simulink model "HostOfSeal"  (R2025a)
settings: Solver=FixedStepDiscrete  StartTime=0.0  StopTime=30  FixedStep=0.025  RelTol=1e-3
model workspace (MATLAB code in the model file + MAT data in the model file):
  | cmdLim = Simulink.Parameter;
  | cmdLim.Value = 15;
  | cmdLim.Description = 'Limit for controlling the maximum surface command angle.';
  | cmdLim.Min = 0;
  | cmdLim.Max = 90;
  | cmdLim.DocUnits = 'deg';
  | 
  | dispGain = Simulink.Parameter;
  | dispGain.Value = 0.75;
  | dispGain.Description = 'Gain applied to the displacement error.';
  | dispGain.Min = 0;
  | dispGain.Max = [];
  | dispGain.DocUnits = 'deg/sec/deg';
  | 
  | dispLim = Simulink.Parameter;
  | dispLim.Value = 30;
  | dispLim.Description = 'Limit for controlling the maximum commanded angle.';
  | dispLim.Min = 0;
  | dispLim.Max = 180;
  | dispLim.DocUnits = 'deg';
  | 
  | intGain = Simulink.Parameter;
  | intGain.Value = 0.5;
  | intGain.Description = 'Gain applied to the integral error.';
  | intGain.Min = 0;
  | intGain.Max = [];
  | intGain.DocUnits = 'deg/sec/deg/sec';
  | 
  | intLim = Simulink.Parameter;
  | intLim.Value = 5;
  | intLim.Description = 'Limit for controlling the maximum commanded angle.';
  | intLim.Min = 0;
  | intLim.Max = 90;
  | intLim.DocUnits = 'deg';
  | 
  | rateGain = Simulink.Parameter;
  | rateGain.Value = 2;
  | rateGain.Description = 'Gain applied to the rate error.';
  | rateGain.Min = 0;
  | rateGain.Max = [];
  | rateGain.DocUnits = 'deg/deg/sec';
  | 
  | rateLim = Simulink.Parameter;
  | rateLim.Value = 6;
  | rateLim.Description = 'Limit for controlling the maximum commanded angle.';
  | rateLim.Min = 0;
  | rateLim.Max = 180;
  | rateLim.DocUnits = 'deg/sec';
  | 
  | hdgGain = Simulink.Parameter;
  | hdgGain.Value = 0.015;
values from neighbouring files (symbols this model uses):
  DriveTs = 100e-6    (= 0.0001)    [simpars.m]
  Jm = 1    [simpars.m]
  KEp = Kt * sqrt(2) / 1.5    [simpars.m]
  Kt = 1    [simpars.m]
  Lm = 1e-3    (= 0.001)    [simpars.m]
  PolePairs = 5    [simpars.m]
  Rm = 1    [simpars.m]
  Vdc = 24    [simpars.m]
undefined symbols (not defined in the file or in its folder): CurrentCommand, DcBusVoltage, EncoderMain, EncoderMainSpeed, Iq, KiSpeed, Kp, KpSpeed, PositionCommand, SpeedCommand, SystemTime
libraries: simulink x1
(part 1 of 2)
Description:
  | This model represents a basic roll axis autopilot with two operating
  | modes; roll attitude hold and heading hold. The mode logic for these
  | modes is external to this model.  The model architecture represents the
  | heading hold mode and basic roll attitude function as referenced models.
  | 
  | The roll attitude control function is a PID controller that uses roll
  | attitude and roll rate feedback to produce an aileron command.  The
  | input to the controller will be either a basic roll angle reference or a
  | roll command to track the desired heading.
settings Model: RequirementInfo={} %GIDa_fe9045fd_0412_4b6e_8206_617cc20e6fde  DataDictionary=SEALGenericTypes_1.sldd  FPTRunName=Active  ModifiedByFormat=The MathWorks, Inc.  Creator=The MathWorks, Inc.  LastModifiedBy=The MathWorks, Inc.
settings SolverCC: AlgebraicLoopSolver=TrustRegion
settings DataIOCC: ExternalInput=xin  SaveFormat=StructureWithTime  SaveOutput=off  SignalLogging=off  DSMLogging=off  SaveTime=off  ReturnWorkspaceOutputs=off
settings OptimizationCC: DefaultParameterBehavior=Inlined  UseDivisionForNetSlopeComputation=on  UseFloatMulNetSlope=on  InlineInvariantSignals=on  ReuseModelBlockBuffer=off  EnhancedBackFolding=on  BooleansAsBitfields=on  PassReuseOutputArgsAs=Individual arguments  ExpressionDepthLimit=2147483647.0  StateBitsets=on  DataBitsets=on  ZeroExternalMemoryAtStartup=off  ZeroInternalMemoryAtStartup=off  NoFixptDivByZeroProtection=on  EfficientFloat2IntCast=on  LifeSpan=inf  MaxStackSize=inf  EfficientTunableParamExpr=on
settings DebuggingCC: SignalRangeChecking=error  ReadBeforeWriteMsg=EnableAllAsError  WriteAfterWriteMsg=EnableAllAsError  WriteAfterReadMsg=EnableAllAsError  AlgebraicLoopMsg=error  ArtificialAlgebraicLoopMsg=error  SaveWithDisabledLinksMsg=error  SaveWithParameterizedLinksMsg=error  CheckExecutionContextPreStartOutputMsg=on  BlockPriorityViolationMsg=error  MaxConsecutiveZCsMsg=warning  SolverPrmCheckMsg=error  InheritedTsInSrcMsg=error  SingleTaskRateTransMsg=error  TasksWithSamePriorityMsg=error  SigSpecEnsureSampleTimeMsg=error  IntegerOverflowMsg=error  ParameterUnderflowMsg=error  ParameterPrecisionLossMsg=none  ParameterTunabilityLossMsg=error  UnderSpecifiedDataTypeMsg=error  UnnecessaryDatatypeConvMsg=warning  VectorMatrixConversionMsg=error  SignalLabelMismatchMsg=error  UnconnectedInputMsg=error  UnconnectedOutputMsg=error  UnconnectedLineMsg=error  SFcnCompatibilityMsg=error  UniqueDataStoreMsg=error  BusObjectLabelMismatch=error  RootOutportRequireBusObject=error  AssertControl=DisableAll  AllowSymbolicDim=off  ModelReferenceIOMismatchMessage=error  UnknownTsInhSupMsg=error  ModelReferenceDataLoggingMessage=error  ModelReferenceSymbolNameMessage=none  StateNameClashWarn=warning  StrictBusMsg=ErrorOnBusTreatedAsVector  NonBusSignalsTreatedAsBus=error  SFInvalidInputDataAccessInChartInitDiag=error  SFTransitionOutsideNaturalParentDiag=error  SFUnreachableExecutionPathDiag=error  SFUndirectedBroadcastEventsDiag=error  SFExecutionAtInitializationDiag=none  IntegerSaturationMsg=error  ArithmeticOperatorsInVariantConditions=warning
settings HardwareCC: ProdBitPerChar=16.0  ProdBitPerInt=16.0  ProdBitPerPointer=32.0  ProdBitPerSizeT=32.0  ProdBitPerPtrDiffT=32.0  ProdLargestAtomicInteger=Integer  ProdLargestAtomicFloat=None  ProdWordSize=16.0  ProdHWDeviceType=Texas Instruments->C2000  TargetHWDeviceType=32-bit Generic
settings ModelReferenceCC: EnableRefExpFcnMdlSchedulingChecks=on  ModelReferenceNumInstancesAllowed=Single  PropagateSignalLabelsOutOfModel=off
settings SFSimCC: SimUseLocalCustomCode=off  MATLABDynamicMemAlloc=off
settings SFSimCC: SimCustomHeaderCode=|
  | #include "CANServer.h"
  | #include "DeviceSetup.h"
settings SFSimCC: SimUserSources=|
  | .\ExternalCode\CANServer.c
  | .\ExternalCode\DeviceSetup.c
settings RTWCC: SystemTargetFile=ert.tlc  GenCodeOnly=on  TemplateMakefile=ert_default_tmf  PostCodeGenCommand=PrepWrapper  GenerateReport=on  RTWVerbose=off  RTWUseLocalCustomCode=off  RTWUseSimCustomCode=on  BuildConfiguration=Faster Runs  IncludeHyperlinkInReport=on  LaunchReport=on  GenerateTraceInfo=on  GenerateTraceReport=on  GenerateTraceReportSl=on  GenerateTraceReportSf=on  GenerateTraceReportEml=on  GenerateCodeMetricsReport=on  GPUComputeCapability=3.5  DLArmComputeVersion=19.05  Description=Embedded Coder
settings RTWCC: CustomHeaderCode=|
  | #include "CANServer.h"
  | #include "DeviceSetup.h"
settings RTWCC: CustomSource=|
  | .\ExternalCode\CANServer.c
  | .\ExternalCode\DeviceSetup.c
settings CodeAppCC: ForceParamTrailComments=on  IgnoreCustomStorageClasses=off  SimulinkDataObjDesc=on  CustomSymbolStrGlobalVar=rt$N$M  CustomSymbolStrType=$N$M  CustomSymbolStrFcn=$N$M$F  CustomSymbolStrMacro=$N$M  InsertBlockDesc=on  ReqsInCode=on
settings ERTTargetCC: ExtModeTransport=0.0  ExtModeStaticAlloc=off  ExtModeMexFile=ext_comm  ExtModeIntrfLevel=Level1  ERTCustomFileTemplate=example_file_process.tlc  ERTFilePackagingFormat=CompactWithDataFile  ConvertIfToSwitch=off  SuppressUnreachableDefaultCases=off  DynamicArrayContainerType=coder::array  UtilityFuncGeneration=Shared location  MultiwordLength=2048.0  GenerateSampleERTMain=on  IncludeMdlTerminateFcn=off  CombineSignalStateStructs=on  SuppressErrorStatus=on  SupportAbsoluteTime=off  SubcomponentCodeInterfacePackaging=Nonreusable function  SupportNonFinite=off  SupportComplex=off
settings ConfigComp: CovScope=ReferencedModels  CovSaveName=covdata_rollAP  CovMetricSettings=dcmtrwe  CovHTMLOptions=-sRT=1 -aTS=1 -bRG=1 -bTC=1 -hTR=1 -nFC=0 -scm=1 -bcm=1 -xEv=0  CovSaveCumulativeToWorkspaceVar=on  CovSaveSingleToWorkspaceVar=on  CovCumulativeVarName=covCumulativeData_rollAP  CovReportOnPause=off  CovExternalEMLEnable=off  CovSFcnEnable=off  DVMaxProcessTime=300.0  DVModelCoverageObjectives=MCDC  DVMaxTestCaseSteps=500.0  DVTestSuiteOptimization=Auto  DVAbsoluteTolerance=1.0e-5  DVDefectChecker=off  DVDetectActiveLogic=on  DVMaxViolationSteps=20.0  DVSaveHarnessModel=on  DVModelReferenceHarness=on  DVHarnessSource=Signal Editor  DVSaveReport=on  DVRebuildModelRepresentation=Always  DVActiveTab=0.0

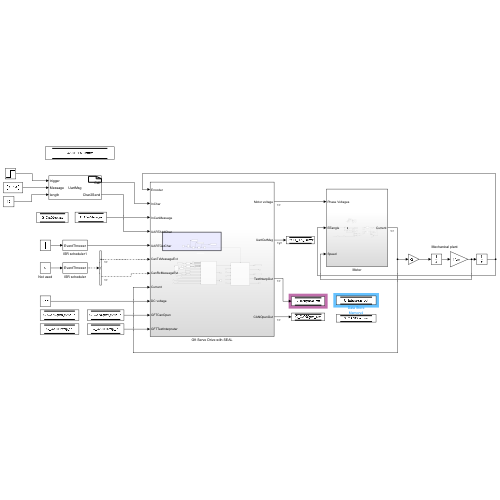
[thumbnail: Simulink's stored preview of the top-level diagram]
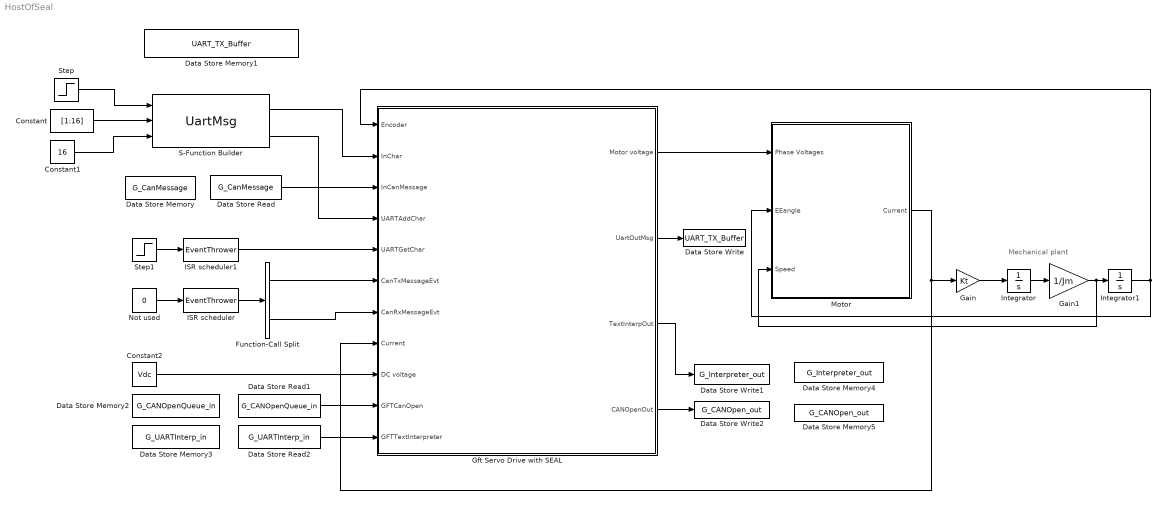
== system HostOfSeal ==
  note: Mechanical plant
  Constant : Constant  Value=[1:16]
  Constant1 : Constant  Value=16
  Constant2 : Constant  Value=Vdc
  Data Store Memory : DataStoreMemory  DataStoreName=G_CanMessage  WriteAfterWriteMsg=warning  InitialValue=CANMessage_Init  ShowAdditionalParam=off  OutDataTypeStr=Bus: CANMessage_T
  Data Store Memory1 : DataStoreMemory  DataStoreName=UART_TX_Buffer  WriteAfterWriteMsg=warning  ShowAdditionalParam=off  OutDataTypeStr=Bus: UartCyclicBuf_T
  Data Store Memory2 : DataStoreMemory  DataStoreName=G_CANOpenQueue_in  WriteAfterWriteMsg=warning  ShowAdditionalParam=off  OutDataTypeStr=Bus: CANCyclicBuf_T
  Data Store Memory3 : DataStoreMemory  DataStoreName=G_UARTInterp_in  WriteAfterWriteMsg=warning  ShowAdditionalParam=off
  Data Store Memory4 : DataStoreMemory  DataStoreName=G_Interpreter_out  WriteAfterWriteMsg=warning  ShowAdditionalParam=off  OutDataTypeStr=Bus: UartCyclicBuf_T
  Data Store Memory5 : DataStoreMemory  DataStoreName=G_CANOpen_out  WriteAfterWriteMsg=warning  ShowAdditionalParam=off  OutDataTypeStr=Bus: CANCyclicBuf_T
  Data Store Read : DataStoreRead  DataStoreName=G_CanMessage  IndexOptions=Index vector (dialog)  Indices=1  OutputSizes=1
  Data Store Read1 : DataStoreRead  DataStoreName=G_CANOpenQueue_in  IndexOptions=Index vector (dialog)  Indices=1  OutputSizes=1
  Data Store Read2 : DataStoreRead  DataStoreName=G_UARTInterp_in  IndexOptions=Index vector (dialog)  Indices=1  OutputSizes=1
  Data Store Write : DataStoreWrite  DataStoreName=UART_TX_Buffer  IndexOptions=Index vector (dialog)  Indices=1  OutputSizes=1
  Data Store Write1 : DataStoreWrite  DataStoreName=G_Interpreter_out  IndexOptions=Index vector (dialog)  Indices=1  OutputSizes=1
  Data Store Write2 : DataStoreWrite  DataStoreName=G_CANOpen_out  IndexOptions=Index vector (dialog)  Indices=1  OutputSizes=1
  Function-Call Split : FunctionCallSplit  IconShape=distinctive  NumOutputPorts=2  OutputPortLayout=default
  Gain : Gain  Gain=Kt
  Gain1 : Gain  Gain=1/Jm
  Gft Servo Drive with SEAL : Subsystem
  ISR scheduler : M-S-Function  FunctionName=EventThrower
  ISR scheduler1 : M-S-Function  FunctionName=EventThrower
  Integrator : Integrator
  Integrator1 : Integrator
  Motor : Subsystem
  Not used : Constant  Value=0
  S-Function Builder : S-Function  FunctionName=UartMsg  SFunctionModules=UartMsg_wrapper.c  SFunctionDeploymentMode=off  EnableBusSupport=off  mask(S-Function Builder){}
      mask help: Simulink:masks:SFunctionBuilder_MD
      mask init:
      | val = [[.9  0.75 0.75 1 1 .9 .9 1]',[1 1 0.75 0.75 .9 .9 1 .9]'];try , sys = get_param(gcb,'SfunBuilderFcnName');if isempty(sys), sys = get_param(gcb,'FunctionName'); end,catch, sys = get_param(gcb,'FunctionName'); end
      settings: CopyFcn=set_param(gcbh,'LinkStatus','none')  OpenFcn=sfunctionwizard(gcbh)
      mask Display:
      | plot(val(:,1),val(:,2))
      | disp(sys)
      | port_label('input',1,sprintf('%s', 'trigger'),'interpreter','tex')
      | port_label('input',2,sprintf('%s', 'Message'),'interpreter','tex')
      | port_label('input',3,sprintf('%s', 'length'),'interpreter','tex')
      | port_label('output',1,sprintf('%s', 'Call'),'interpreter','tex')
      | port_label('output',2,sprintf('%s', 'Char2Send'),'interpreter','tex')
  Step : Step  Time=0.001  SampleTime=0
  Step1 : Step  Time=0.001  SampleTime=0
  wires:
  Constant2/1 -> Gft Servo Drive with SEAL/9(DC voltage)
  Motor/1(Current) -> Gft Servo Drive with SEAL/8(Current), Gain/1
  Gain/1 -> Integrator/1
  Integrator/1 -> Gain1/1
  Gain1/1 -> Motor/3(Speed), Integrator1/1
  Integrator1/1 -> Motor/2(EEangle), Gft Servo Drive with SEAL/1(Encoder)
  Gft Servo Drive with SEAL/1(Motor voltage) -> Motor/1(Phase Voltages)
  Not used/1 -> ISR scheduler/1
  ISR scheduler/1 -> Function-Call Split/1
  Data Store Read/1 -> Gft Servo Drive with SEAL/3(InCanMessage)
  Function-Call Split/1 -> Gft Servo Drive with SEAL/6(CanTxMessageEvt)
  Function-Call Split/2 -> Gft Servo Drive with SEAL/7(CanRxMessageEvt)
  S-Function Builder/1 -> Gft Servo Drive with SEAL/2(InChar)
  S-Function Builder/2 -> Gft Servo Drive with SEAL/4(UARTAddChar)
  Constant/1 -> S-Function Builder/2
  Constant1/1 -> S-Function Builder/3
  Step/1 -> S-Function Builder/1
  ISR scheduler1/1 -> Gft Servo Drive with SEAL/5(UARTGetChar)
  Step1/1 -> ISR scheduler1/1
  Gft Servo Drive with SEAL/2(UartOutMsg) -> Data Store Write/1
  Data Store Read1/1 -> Gft Servo Drive with SEAL/10(GFTCanOpen)
  Data Store Read2/1 -> Gft Servo Drive with SEAL/11(GFTTextInterpreter)
  Gft Servo Drive with SEAL/3(TextInterpOut) -> Data Store Write1/1
  Gft Servo Drive with SEAL/4(CANOpenOut) -> Data Store Write2/1

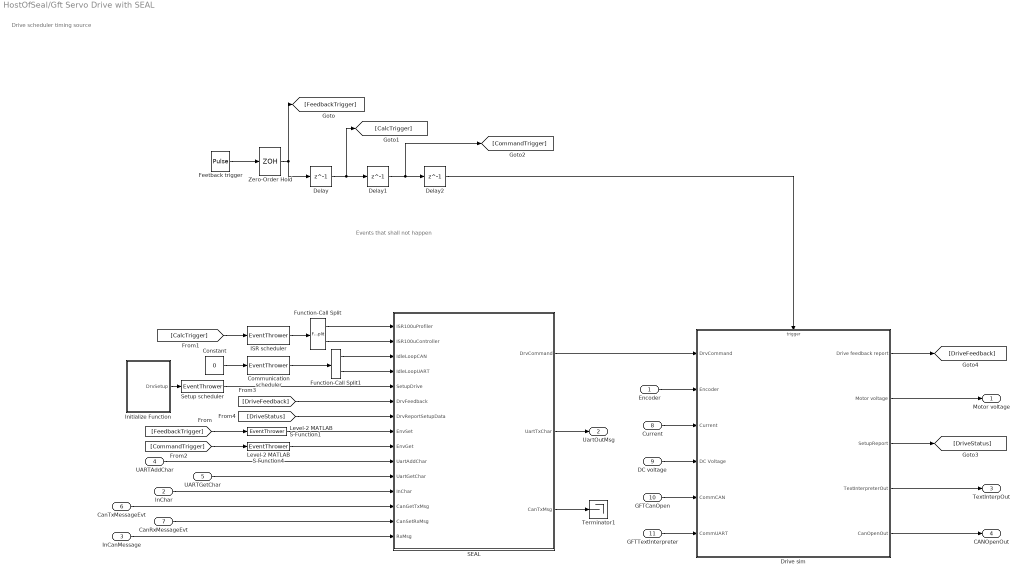
== system HostOfSeal/Gft Servo Drive with SEAL ==
  note: Drive scheduler timing source
  note: Events that shall not happen
  Encoder : Inport
  InChar : Inport  Port=2
  InCanMessage : Inport  Port=3
  UARTAddChar : Inport  Priority=1  Port=4  PortDimensions=1  OutputFunctionCall=on
  UARTGetChar : Inport  Priority=1  Port=5  PortDimensions=1  OutputFunctionCall=on
  CanTxMessageEvt : Inport  Priority=1  Port=6  PortDimensions=1  OutputFunctionCall=on
  CanRxMessageEvt : Inport  Priority=1  Port=7  PortDimensions=1  OutputFunctionCall=on
  Current : Inport  Port=8
  DC voltage : Inport  Port=9
  GFTCanOpen : Inport  Port=10
  GFTTextInterpreter : Inport  Port=11
  Communication scheduler : M-S-Function  FunctionName=EventThrower
  Constant : Constant  Value=0
  Delay : Delay  DelayLength=1  InitialCondition=0  SampleTime=DriveTs/4
  Delay1 : Delay  DelayLength=1  InitialCondition=0  SampleTime=DriveTs/4
  Delay2 : Delay  DelayLength=1  InitialCondition=0  SampleTime=DriveTs/4
  Drive sim : Subsystem  TreatAsAtomicUnit=on
  Feetback trigger : DiscretePulseGenerator  PulseType=Time based  Period=DriveTs  PulseWidth=5
  Function-Call Split : FunctionCallSplit  IconShape=distinctive  NumOutputPorts=2  OutputPortLayout=default
  Function-Call Split1 : FunctionCallSplit  IconShape=distinctive  NumOutputPorts=2  OutputPortLayout=default
  ISR scheduler : M-S-Function  FunctionName=EventThrower
  Initialize Function : Subsystem  TreatAsAtomicUnit=on
  Level-2 MATLAB S-Function1 : M-S-Function  FunctionName=EventThrower
  Level-2 MATLAB S-Function4 : M-S-Function  FunctionName=EventThrower
  SEAL : Subsystem
  Setup scheduler : M-S-Function  FunctionName=EventThrower
  Terminator1 : Terminator
  Zero-Order Hold : ZeroOrderHold  SampleTime=DriveTs/4
  Motor voltage : Outport
  UartOutMsg : Outport  Port=2
  TextInterpOut : Outport  Port=3
  CANOpenOut : Outport  Port=4
  wires:
  Communication scheduler/1 -> Function-Call Split1/1
  Delay/1 -> [CalcTrigger], Delay1/1
  Delay1/1 -> [CommandTrigger], Delay2/1
  Drive sim/2(Motor voltage) -> Motor voltage/1
  Zero-Order Hold/1 -> [FeedbackTrigger], Delay/1
  [FeedbackTrigger] -> Level-2 MATLAB S-Function1/1
  Delay2/1 -> Drive sim/Trigger
  Drive sim/1(Drive feedback report) -> [DriveFeedback]
  [CalcTrigger] -> ISR scheduler/1
  [CommandTrigger] -> Level-2 MATLAB S-Function4/1
  Initialize Function/1(DrvSetup) -> Setup scheduler/1
  ISR scheduler/1 -> Function-Call Split/1
  Feetback trigger/1 -> Zero-Order Hold/1
  Constant/1 -> Communication scheduler/1
  Encoder/1 -> Drive sim/2(Encoder)
  Function-Call Split/2 -> SEAL/2(ISR100uController)
  Function-Call Split/1 -> SEAL/1(ISR100uProfiler)
  Function-Call Split1/2 -> SEAL/4(IdleLoopUART)
  Function-Call Split1/1 -> SEAL/3(IdleLoopCAN)
  [DriveFeedback] -> SEAL/6(DrvFeedback)
  [DriveStatus] -> SEAL/7(DrvReportSetupData)
  Setup scheduler/1 -> SEAL/5(SetupDrive)
  SEAL/2(UartTxChar) -> UartOutMsg/1
  SEAL/3(CanTxMsg) -> Terminator1/1
  Level-2 MATLAB S-Function1/1 -> SEAL/8(EnvSet)
  Level-2 MATLAB S-Function4/1 -> SEAL/9(EnvGet)
  InChar/1 -> SEAL/12(InChar)
  InCanMessage/1 -> SEAL/15(RxMsg)
  UARTAddChar/1 -> SEAL/10(UartAddChar)
  UARTGetChar/1 -> SEAL/11(UartGetChar)
  CanTxMessageEvt/1 -> SEAL/13(CanGetTxMsg)
  CanRxMessageEvt/1 -> SEAL/14(CanSetRxMsg)
  Current/1 -> Drive sim/3(Current)
  DC voltage/1 -> Drive sim/4(DC Voltage)
  Drive sim/3(SetupReport) -> [DriveStatus]
  SEAL/1(DrvCommand) -> Drive sim/1(DrvCommand)
  GFTCanOpen/1 -> Drive sim/5(CommCAN)
  GFTTextInterpreter/1 -> Drive sim/6(CommUART)
  Drive sim/4(TextInterpreterOut) -> TextInterpOut/1
  Drive sim/5(CanOpenOut) -> CANOpenOut/1

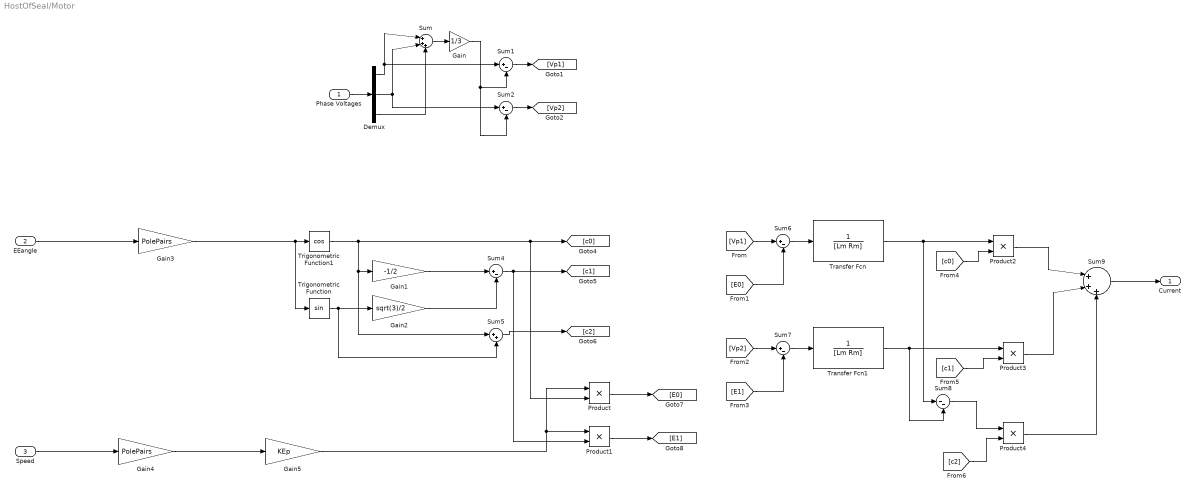
== system HostOfSeal/Motor ==
  Phase Voltages : Inport
  EEangle : Inport  Port=2
  Speed : Inport  Port=3
  Demux : Demux  Outputs=3
  Gain : Gain  Gain=1/3
  Gain1 : Gain  Gain=-1/2
  Gain2 : Gain  Gain=sqrt(3)/2
  Gain3 : Gain  Gain=PolePairs
  Gain4 : Gain  Gain=PolePairs
  Gain5 : Gain  Gain=KEp
  Product{,1..4} (5 alike) : Product
  Sum : Sum  Inputs=|+++
  Sum{1..2,4,6..7} (5 alike) : Sum  Inputs=|+-
  Sum5 : Sum  Inputs=|++
  Sum8 : Sum  Inputs=|--
  Sum9 : Sum  Inputs=|+++
  Transfer Fcn : TransferFcn  Denominator=[Lm Rm]
  Transfer Fcn1 : TransferFcn  Denominator=[Lm Rm]
  Trigonometric Function : Trigonometry
  Trigonometric Function1 : Trigonometry  Operator=cos
  Current : Outport
  wires:
  Phase Voltages/1 -> Demux/1
  Demux/3 -> Sum/3
  Demux/2 -> Sum/2, Sum2/1
  Demux/1 -> Sum1/1, Sum/1
  Sum/1 -> Gain/1
  Gain/1 -> Sum2/2, Sum1/2
  Sum1/1 -> [Vp1]
  Sum2/1 -> [Vp2]
  EEangle/1 -> Gain3/1
  Trigonometric Function1/1 -> Sum5/1, Gain1/1, Product/2, [c0]
  Trigonometric Function/1 -> Sum5/2, Gain2/1
  Gain1/1 -> Sum4/1
  Gain2/1 -> Sum4/2
  Sum4/1 -> Product1/2, [c1]
  Sum5/1 -> [c2]
  Gain3/1 -> Trigonometric Function/1, Trigonometric Function1/1
  Speed/1 -> Gain4/1
  Gain4/1 -> Gain5/1
  Product/1 -> [E0]
  Product1/1 -> [E1]
  [Vp1] -> Sum6/1
  [E0] -> Sum6/2
  Sum6/1 -> Transfer Fcn/1
  Sum7/1 -> Transfer Fcn1/1
  [Vp2] -> Sum7/1
  [E1] -> Sum7/2
  Transfer Fcn1/1 -> Product3/1, Sum8/2
  Transfer Fcn/1 -> Sum8/1, Product2/1
  Sum8/1 -> Product4/1
  [c0] -> Product2/2
  [c1] -> Product3/2
  [c2] -> Product4/2
  Product2/1 -> Sum9/1
  Product3/1 -> Sum9/2
  Product4/1 -> Sum9/3
  Sum9/1 -> Current/1
  Gain5/1 -> Product1/1, Product/1

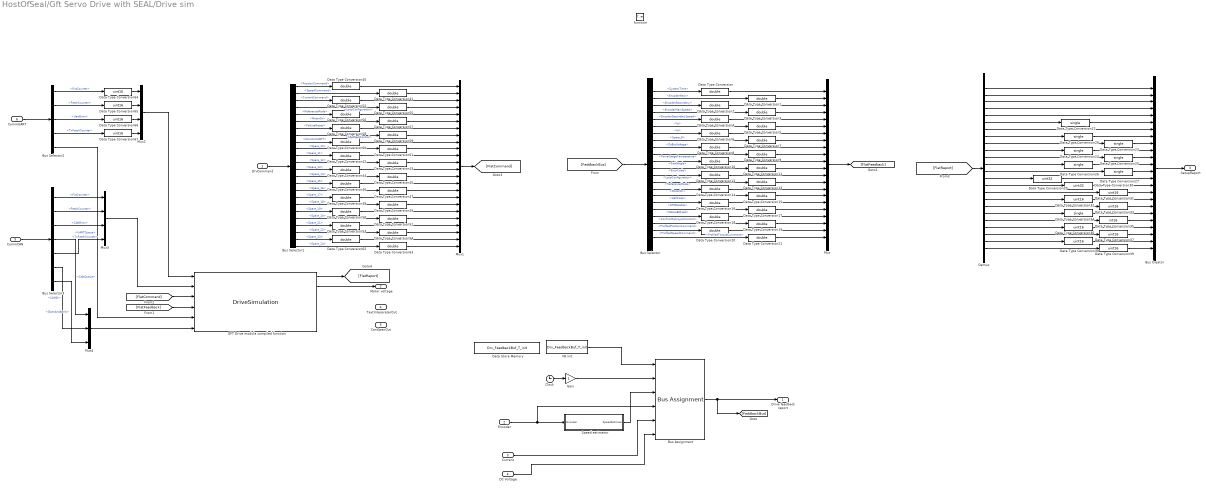
== system HostOfSeal/Gft Servo Drive with SEAL/Drive sim ==
  DrvCommand : Inport  OutDataTypeStr=Bus: DrvCommandBuf_T
  Encoder : Inport  Port=2
  Current : Inport  Port=3
  DC Voltage : Inport  Port=4
  CommCAN : Inport  Port=5  OutDataTypeStr=Bus: CANCyclicBuf_T
  CommUART : Inport  Port=6  OutDataTypeStr=Bus: UartCyclicBuf_T
  function : TriggerPort  TriggerType=function-call  VariantControl=(inherit)
  Bus Assignment : BusAssignment  AssignedSignals=SystemTime,EncoderMainSpeed,EncoderMain,Iq,DcBusVoltage
  Bus Creator : BusCreator  Inputs=24  OutDataTypeStr=Bus: SetupReportBuf_T  NonVirtualBus=on
      settings: AttributesFormatString=%<ShowName>  InheritFromInputs=off
  Bus Selector : BusSelector  OutputSignals=SystemTime,EncoderMain,EncoderSecondary,EncoderMainSpeed,EncoderSecondarySpeed,Iq,Id,Spare_8,DcBusVoltage,PowerStageTemperature,FieldAngle,ErrorCode,LoopConfiguration,ReferenceMode,MotorOn,HallCode,STODisable,StatusBitField,ConfirmRelinquishControl,ProfiledPositionCommand,ProfiledSpeedCommand,ProfiledTorqueCommand
  Bus Selector1 : BusSelector  OutputSignals=PositionCommand,SpeedCommand,CurrentCommand,LoopConfiguration,ReferenceMode,MotorOn,FailureReset,bSetSealControl,bControlUART,Spare_10,Spare_11,Spare_12,Spare_13,Spare_14,Spare_15,Spare_16,Spare_17,Spare_18,Spare_19,Spare_20,Spare_21,Spare_22,Spare_23,Spare_24
  Bus Selector2 : BusSelector  OutputSignals=PutCounter,FetchCounter,UartError,TxFetchCounter,UARTQueue
  Bus Selector3 : BusSelector  OutputSignals=PutCounter,FetchCounter,CANError,CANQueue,TxFetchCounter,CANID,DLenAndAttrib
  Clock : Clock
  Data Store Memory : DataStoreMemory  DataStoreName=Drv_FeedbackBuf_T_init  WriteAfterWriteMsg=warning  InitialValue=Drv_FeedbackBuf_T_init  ShowAdditionalParam=off  OutDataTypeStr=Bus: FeedbackBuf_T
  Data Type Conversion{,1..21,40..63} (46 alike) : DataTypeConversion  OutDataTypeStr=double  SaturateOnIntegerOverflow=off  RndMeth=Floor
  Data Type Conversion{22..28,34} (8 alike) : DataTypeConversion  OutDataTypeStr=single  SaturateOnIntegerOverflow=off  RndMeth=Floor
  Data Type Conversion29 : DataTypeConversion  OutDataTypeStr=uint32  SaturateOnIntegerOverflow=off  RndMeth=Floor
  Data Type Conversion30 : DataTypeConversion  OutDataTypeStr=uint32  SaturateOnIntegerOverflow=off  RndMeth=Floor
  Data Type Conversion{31..33,36..39,64..67} (11 alike) : DataTypeConversion  OutDataTypeStr=uint16  SaturateOnIntegerOverflow=off  RndMeth=Floor
  Data Type Conversion35 : DataTypeConversion  OutDataTypeStr=int16  SaturateOnIntegerOverflow=off  RndMeth=Floor
  Demux : Demux  Outputs=24
  FB init : DataStoreRead  DataStoreName=Drv_FeedbackBuf_T_init  IndexOptions=Index vector (dialog)  Indices=1  OutputSizes=1
  GFT Drive module compiled function : S-Function  FunctionName=DriveSimulation  SFunctionModules=DriveSimulation_wrapper.c  SFunctionDeploymentMode=off  EnableBusSupport=off  mask(S-Function Builder){}
      mask help: Simulink:masks:SFunctionBuilder_MD
      mask init: same as HostOfSeal/S-Function Builder
      settings: CopyFcn=set_param(gcbh,'LinkStatus','none')  OpenFcn=sfunctionwizard(gcbh)
      mask Display:
      | plot(val(:,1),val(:,2))
      | disp(sys)
      | port_label('input',1,sprintf('%s', 'UARTManagement\_in'),'interpreter','tex')
      | port_label('input',2,sprintf('%s', 'CANManagement\_in'),'interpreter','tex')
      | port_label('input',3,sprintf('%s', 'DrvCommand'),'interpreter','tex')
      | port_label('input',4,sprintf('%s', 'Feedback'),'interpreter','tex')
      | port_label('input',5,sprintf('%s', 'UARTBuffer\_in'),'interpreter','tex')
      | port_label('input',6,sprintf('%s', 'CANBuffer\_in'),'interpreter','tex')
      | port_label('output',1,sprintf('%s', 'SetupReport'),'interpreter','tex')
      | port_label('output',2,sprintf('%s', 'PhaseVoltages'),'interpreter','tex')
      | port_label('output',3,sprintf('%s', 'TextInterpOutManagement'),'interpreter','tex')
      | port_label('output',4,sprintf('%s', 'TextInterpBuffer'),'interpreter','tex')
      | port_label('output',5,sprintf('%s', 'CanOpenManagement\_out'),'interpreter','tex')
      | port_label('output',6,sprintf('%s', 'CanOpenBufferOut'),'interpreter','tex')
  Gain : Gain
  Mux : Mux  Inputs=22
  Mux1 : Mux  Inputs=24
  Mux2 : Mux
  Mux3 : Mux
  Mux4 : Mux  Inputs=3
  Speed estimator : Subsystem
  Drive feedback report : Outport  OutDataTypeStr=Bus: FeedbackBuf_T
  Motor voltage : Outport  Port=2
  SetupReport : Outport  Port=3
  TextInterpreterOut : Outport  Port=4
  CanOpenOut : Outport  Port=5
  wires:
  Clock/1 -> Gain/1
  FB init/1 -> Bus Assignment/1
  Bus Assignment/1 -> [FeddbackBus], Drive feedback report/1
  Gain/1 -> Bus Assignment/2
  Encoder/1 -> Bus Assignment/4, Speed estimator/1(Encoder)
  Speed estimator/1(SpeedEstimae) -> Bus Assignment/3
  Current/1 -> Bus Assignment/5
  DC Voltage/1 -> Bus Assignment/6
  [FeddbackBus] -> Bus Selector/1
  Bus Selector/1 -> Data Type Conversion/1  "<SystemTime>"
  Bus Selector/2 -> Data Type Conversion1/1  "<EncoderMain>"
  Bus Selector/3 -> Data Type Conversion2/1  "<EncoderSecondary>"
  Bus Selector/4 -> Data Type Conversion3/1  "<EncoderMainSpeed>"
  Bus Selector/6 -> Data Type Conversion5/1  "<Iq>"
  Bus Selector/7 -> Data Type Conversion6/1  "<Id>"
  Bus Selector/5 -> Data Type Conversion4/1  "<EncoderSecondarySpeed>"
  Bus Selector/8 -> Data Type Conversion7/1  "<Spare_8>"
  Bus Selector/9 -> Data Type Conversion8/1  "<DcBusVoltage>"
  Bus Selector/10 -> Data Type Conversion9/1  "<PowerStageTemperature>"
  Bus Selector/11 -> Data Type Conversion10/1  "<FieldAngle>"
  Bus Selector/12 -> Data Type Conversion11/1  "<ErrorCode>"
  Bus Selector/13 -> Data Type Conversion12/1  "<LoopConfiguration>"
  Bus Selector/14 -> Data Type Conversion13/1  "<ReferenceMode>"
  Bus Selector/15 -> Data Type Conversion14/1  "<MotorOn>"
  Bus Selector/16 -> Data Type Conversion15/1  "<HallCode>"
  Bus Selector/17 -> Data Type Conversion16/1  "<STODisable>"
  Bus Selector/18 -> Data Type Conversion17/1  "<StatusBitField>"
  Bus Selector/19 -> Data Type Conversion18/1  "<ConfirmRelinquishControl>"
  Bus Selector/20 -> Data Type Conversion19/1  "<ProfiledPositionCommand>"
  Bus Selector/21 -> Data Type Conversion20/1  "<ProfiledSpeedCommand>"
  Bus Selector/22 -> Data Type Conversion21/1  "<ProfiledTorqueCommand>"
  Data Type Conversion/1 -> Mux/1
  Data Type Conversion1/1 -> Mux/2
  Data Type Conversion2/1 -> Mux/3
  Data Type Conversion3/1 -> Mux/4
  Data Type Conversion4/1 -> Mux/5
  Data Type Conversion5/1 -> Mux/6
  Data Type Conversion6/1 -> Mux/7
  Data Type Conversion7/1 -> Mux/8
  Data Type Conversion8/1 -> Mux/9
  Data Type Conversion9/1 -> Mux/10
  Data Type Conversion10/1 -> Mux/11
  Data Type Conversion11/1 -> Mux/12
  Data Type Conversion12/1 -> Mux/13
  Data Type Conversion13/1 -> Mux/14
  Data Type Conversion14/1 -> Mux/15
  Data Type Conversion15/1 -> Mux/16
  Data Type Conversion16/1 -> Mux/17
  Data Type Conversion17/1 -> Mux/18
  Data Type Conversion18/1 -> Mux/19
  Data Type Conversion19/1 -> Mux/20
  Data Type Conversion20/1 -> Mux/21
  Data Type Conversion21/1 -> Mux/22
  Mux/1 -> [FlatFeedback]
  Demux/3 -> Bus Creator/3
  Demux/4 -> Bus Creator/4
  Demux/5 -> Bus Creator/5
  Demux/2 -> Bus Creator/2
  Demux/7 -> Bus Creator/7
  Demux/8 -> Data Type Conversion28/1
  Demux/9 -> Data Type Conversion23/1
  Demux/10 -> Data Type Conversion24/1
  Demux/11 -> Data Type Conversion25/1
  Demux/12 -> Data Type Conversion26/1
  Demux/13 -> Data Type Conversion27/1
  Demux/14 -> Data Type Conversion29/1
  Demux/15 -> Data Type Conversion30/1
  Demux/16 -> Data Type Conversion31/1
  Demux/17 -> Data Type Conversion32/1
  Demux/18 -> Data Type Conversion33/1
  Demux/20 -> Data Type Conversion35/1
  Demux/19 -> Data Type Conversion34/1
  Demux/21 -> Data Type Conversion36/1
  Demux/23 -> Data Type Conversion38/1
  Demux/24 -> Data Type Conversion39/1
  Demux/22 -> Data Type Conversion37/1
  Demux/1 -> Bus Creator/1
  Demux/6 -> Data Type Conversion22/1
  Data Type Conversion22/1 -> Bus Creator/6
  Data Type Conversion23/1 -> Bus Creator/9
  Data Type Conversion24/1 -> Bus Creator/10
  Data Type Conversion25/1 -> Bus Creator/11
  Data Type Conversion26/1 -> Bus Creator/12
  Data Type Conversion27/1 -> Bus Creator/13
  Data Type Conversion28/1 -> Bus Creator/8
  Data Type Conversion29/1 -> Bus Creator/14
  Data Type Conversion30/1 -> Bus Creator/15
  Data Type Conversion31/1 -> Bus Creator/16
  Data Type Conversion32/1 -> Bus Creator/17
  Data Type Conversion33/1 -> Bus Creator/18
  Data Type Conversion34/1 -> Bus Creator/19
  Data Type Conversion35/1 -> Bus Creator/20
  Data Type Conversion36/1 -> Bus Creator/21
  Data Type Conversion37/1 -> Bus Creator/22
  Data Type Conversion38/1 -> Bus Creator/23
  Data Type Conversion39/1 -> Bus Creator/24
  Bus Creator/1 -> SetupReport/1
  DrvCommand/1 -> Bus Selector1/1
  Data Type Conversion59/1 -> Mux1/8
  Data Type Conversion55/1 -> Mux1/4
  Data Type Conversion56/1 -> Mux1/5
  Data Type Conversion51/1 -> Mux1/20
  Data Type Conversion45/1 -> Mux1/14
  Data Type Conversion50/1 -> Mux1/19
  Data Type Conversion61/1 -> Mux1/10
  Data Type Conversion57/1 -> Mux1/6
  Data Type Conversion60/1 -> Mux1/9
  Data Type Conversion42/1 -> Mux1/11
  Data Type Conversion48/1 -> Mux1/17
  Data Type Conversion43/1 -> Mux1/12
  Data Type Conversion44/1 -> Mux1/13
  Data Type Conversion53/1 -> Mux1/21
  Data Type Conversion58/1 -> Mux1/7
  Data Type Conversion49/1 -> Mux1/18
  Data Type Conversion46/1 -> Mux1/15
  Data Type Conversion52/1 -> Mux1/3
  Data Type Conversion40/1 -> Mux1/1
  Data Type Conversion54/1 -> Mux1/22
  Data Type Conversion47/1 -> Mux1/16
  Data Type Conversion41/1 -> Mux1/2
  Bus Selector1/1 -> Data Type Conversion40/1  "<PositionCommand>"
  Bus Selector1/3 -> Data Type Conversion52/1  "<CurrentCommand>"
  Bus Selector1/5 -> Data Type Conversion56/1  "<ReferenceMode>"
  Bus Selector1/7 -> Data Type Conversion58/1  "<FailureReset>"
  Bus Selector1/9 -> Data Type Conversion60/1  "<bControlUART>"
  Bus Selector1/11 -> Data Type Conversion42/1  "<Spare_11>"
  Bus Selector1/13 -> Data Type Conversion44/1  "<Spare_13>"
  Bus Selector1/15 -> Data Type Conversion46/1  "<Spare_15>"
  Bus Selector1/17 -> Data Type Conversion48/1  "<Spare_17>"
  Bus Selector1/19 -> Data Type Conversion50/1  "<Spare_19>"
  Bus Selector1/21 -> Data Type Conversion53/1  "<Spare_21>"
  Bus Selector1/2 -> Data Type Conversion41/1  "<SpeedCommand>"
  Bus Selector1/4 -> Data Type Conversion55/1  "<LoopConfiguration>"
  Bus Selector1/6 -> Data Type Conversion57/1  "<MotorOn>"
  Bus Selector1/8 -> Data Type Conversion59/1  "<bSetSealControl>"
  Bus Selector1/10 -> Data Type Conversion61/1  "<Spare_10>"
  Bus Selector1/12 -> Data Type Conversion43/1  "<Spare_12>"
  Bus Selector1/14 -> Data Type Conversion45/1  "<Spare_14>"
  Bus Selector1/16 -> Data Type Conversion47/1  "<Spare_16>"
  Bus Selector1/18 -> Data Type Conversion49/1  "<Spare_18>"
  Bus Selector1/20 -> Data Type Conversion51/1  "<Spare_20>"
  Bus Selector1/22 -> Data Type Conversion54/1  "<Spare_22>"
  Data Type Conversion63/1 -> Mux1/24
  Data Type Conversion62/1 -> Mux1/23
  Bus Selector1/23 -> Data Type Conversion62/1  "<Spare_23>"
  Bus Selector1/24 -> Data Type Conversion63/1  "<Spare_24>"
  [FlatFeedback] -> GFT Drive module compiled function/4
  Mux1/1 -> [FlatCommand]
  [FlatCommand] -> GFT Drive module compiled function/3
  GFT Drive module compiled function/2 -> Motor voltage/1
  GFT Drive module compiled function/1 -> [FlatReport]
  [FlatReport] -> Demux/1
  CommUART/1 -> Bus Selector2/1
  Bus Selector2/1 -> Data Type Conversion64/1  "<PutCounter>"
  Bus Selector2/2 -> Data Type Conversion65/1  "<FetchCounter>"
  Bus Selector2/3 -> Data Type Conversion66/1  "<UartError>"
  Bus Selector2/4 -> Data Type Conversion67/1  "<TxFetchCounter>"
  Data Type Conversion64/1 -> Mux2/1
  Data Type Conversion65/1 -> Mux2/2
  Data Type Conversion66/1 -> Mux2/3
  Data Type Conversion67/1 -> Mux2/4
  Mux2/1 -> GFT Drive module compiled function/1
  Bus Selector2/5 -> GFT Drive module compiled function/5  "<UARTQueue>"
  CommCAN/1 -> Bus Selector3/1
  Bus Selector3/1 -> Mux3/1  "<PutCounter>"
  Bus Selector3/2 -> Mux3/2  "<FetchCounter>"
  Bus Selector3/3 -> Mux3/3  "<CANError>"
  Bus Selector3/5 -> Mux3/4  "<TxFetchCounter>"
  Mux3/1 -> GFT Drive module compiled function/2
  Mux4/1 -> GFT Drive module compiled function/6
  Bus Selector3/7 -> Mux4/3  "<DLenAndAttrib>"
  Bus Selector3/6 -> Mux4/2  "<CANID>"
  Bus Selector3/4 -> Mux4/1  "<CANQueue>"

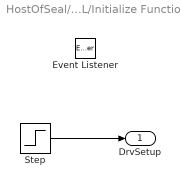
== system HostOfSeal/Gft Servo Drive with SEAL/Initialize Function ==
  Event Listener : EventListener  DisableCoverage=on  EventName=reset
  Step : Step  Time=1e-6  SampleTime=0
  DrvSetup : Outport
  wires:
  Step/1 -> DrvSetup/1

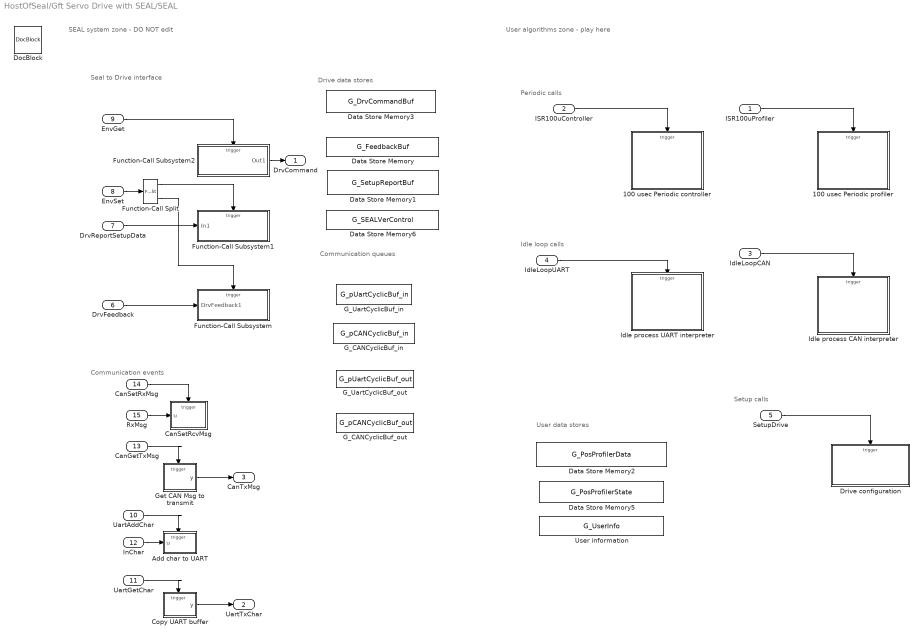
== system HostOfSeal/Gft Servo Drive with SEAL/SEAL ==
  note: User algorithms zone - play here
  note: SEAL system zone - DO NOT edit
  note: Communication events
  note: Idle loop calls
  note: Communication queues
  note: Periodic calls
  note: Seal to Drive interface
  note: Drive data stores
  note: Setup calls
  note: User data stores
  ISR100uProfiler : Inport  Priority=1  OutputFunctionCall=on
  ISR100uController : Inport  Priority=1  Port=2  OutputFunctionCall=on
  IdleLoopCAN : Inport  Priority=1  Port=3  OutputFunctionCall=on
  IdleLoopUART : Inport  Priority=1  Port=4  OutputFunctionCall=on
  SetupDrive : Inport  Priority=1  Port=5  OutputFunctionCall=on
  DrvFeedback : Inport  Port=6  OutDataTypeStr=Bus: FeedbackBuf_T  PortDimensions=1  BusOutputAsStruct=on
  DrvReportSetupData : Inport  Port=7  OutDataTypeStr=Bus: SetupReportBuf_T  PortDimensions=1  BusOutputAsStruct=on
  EnvSet : Inport  Priority=1  Port=8  OutputFunctionCall=on
  EnvGet : Inport  Priority=1  Port=9  OutputFunctionCall=on
  UartAddChar : Inport  Priority=1  Port=10  OutputFunctionCall=on
  UartGetChar : Inport  Priority=1  Port=11  OutputFunctionCall=on
  InChar : Inport  Port=12  PortDimensions=1
  CanGetTxMsg : Inport  Priority=1  Port=13  OutputFunctionCall=on
  CanSetRxMsg : Inport  Priority=1  Port=14  OutputFunctionCall=on
  RxMsg : Inport  Port=15  OutDataTypeStr=Bus: CANMessage_T  PortDimensions=1  BusOutputAsStruct=on
  100 usec Periodic controller : Subsystem  TreatAsAtomicUnit=on
  100 usec Periodic profiler : Subsystem  TreatAsAtomicUnit=on
  Add char to UART : Subsystem  TreatAsAtomicUnit=on
  CanSetRcvMsg : Subsystem  TreatAsAtomicUnit=on
  Copy UART buffer : Subsystem  TreatAsAtomicUnit=on
  Data Store Memory : DataStoreMemory  DataStoreName=G_FeedbackBuf  WriteAfterWriteMsg=warning  VectorParams1D=off  ShowAdditionalParam=off  OutDataTypeStr=Bus: FeedbackBuf_T  StateMustResolveToSignalObject=on
  Data Store Memory1 : DataStoreMemory  DataStoreName=G_SetupReportBuf  WriteAfterWriteMsg=warning  ShowAdditionalParam=off  OutDataTypeStr=Bus: SetupReportBuf_T  StateMustResolveToSignalObject=on
  Data Store Memory2 : DataStoreMemory  DataStoreName=G_PosProfilerData  WriteAfterWriteMsg=warning  InitialValue=PosProfilerData_init  ShowAdditionalParam=off  OutDataTypeStr=Bus: PosProfilerData_T
  Data Store Memory3 : DataStoreMemory  DataStoreName=G_DrvCommandBuf  WriteAfterWriteMsg=warning  ShowAdditionalParam=off  OutDataTypeStr=Bus: DrvCommandBuf_T  StateMustResolveToSignalObject=on
  Data Store Memory5 : DataStoreMemory  DataStoreName=G_PosProfilerState  WriteAfterWriteMsg=warning  InitialValue=PosProfilerState_init  ShowAdditionalParam=off  OutDataTypeStr=Bus: PosProfilerState_T
  Data Store Memory6 : DataStoreMemory  DataStoreName=G_SEALVerControl  WriteAfterWriteMsg=warning  InitialValue=SEALVerControl_init  ShowAdditionalParam=off  OutDataTypeStr=Bus: SEALVerControl_T  StateMustResolveToSignalObject=on
  DocBlock : simulink/Model-Wide Utilities/DocBlock  DocumentType=Text
      content=|
      | These are the global variables for communication with the hosting servo drive.
      | NEVER remove them!
      | They are declared as global variables of the drive.
      | Their structure   is given in the p-coded file HostDriveInterface.p
      |
      | G_DrvCommandBuf     stores the commands to the servo drive.
      | G_SetupReportBuf    reports the setup parameters of the hosting servo drive to the SEAL application
      | FeedbackBuf         reports the feedback and sensor values to the SEAL application.
  Drive configuration : Subsystem  TreatAsAtomicUnit=on
  Function-Call Split : FunctionCallSplit  IconShape=distinctive  NumOutputPorts=2  OutputPortLayout=default
  Function-Call Subsystem : Subsystem  TreatAsAtomicUnit=on
  Function-Call Subsystem1 : Subsystem  TreatAsAtomicUnit=on
  Function-Call Subsystem2 : Subsystem  TreatAsAtomicUnit=on
  G_CANCyclicBuf_in : DataStoreMemory  DataStoreName=G_pCANCyclicBuf_in  WriteAfterWriteMsg=warning  ShowAdditionalParam=off  OutDataTypeStr=Bus: CANCyclicBuf_T  StateMustResolveToSignalObject=on
  G_CANCyclicBuf_out : DataStoreMemory  DataStoreName=G_pCANCyclicBuf_out  WriteAfterWriteMsg=warning  ShowAdditionalParam=off  OutDataTypeStr=Bus: CANCyclicBuf_T  StateMustResolveToSignalObject=on
  G_UartCyclicBuf_in : DataStoreMemory  DataStoreName=G_pUartCyclicBuf_in  WriteAfterWriteMsg=warning  ShowAdditionalParam=off  OutDataTypeStr=Bus: UartCyclicBuf_T  Dimensions=1  StateMustResolveToSignalObject=on
  G_UartCyclicBuf_out : DataStoreMemory  DataStoreName=G_pUartCyclicBuf_out  WriteAfterWriteMsg=warning  ShowAdditionalParam=off  OutDataTypeStr=Bus: UartCyclicBuf_T  StateMustResolveToSignalObject=on
  Get CAN Msg to transmit : Subsystem  TreatAsAtomicUnit=on
  Idle process CAN interpreter : Subsystem  TreatAsAtomicUnit=on
  Idle process UART interpreter : Subsystem  TreatAsAtomicUnit=on
  User information : DataStoreMemory  DataStoreName=G_UserInfo  WriteAfterWriteMsg=warning  InitialValue=G_UserInfo_init  ShowAdditionalParam=off  OutDataTypeStr=Bus: UserInfo_T
  DrvCommand : Outport  OutDataTypeStr=Bus: DrvCommandBuf_T
  UartTxChar : Outport  Port=2  OutDataTypeStr=uint16
  CanTxMsg : Outport  Port=3  OutDataTypeStr=Bus: CANMessage_T  PortDimensions=1
  wires:
  InChar/1 -> Add char to UART/1(u)
  CanSetRxMsg/1 -> CanSetRcvMsg/Trigger
  UartAddChar/1 -> Add char to UART/Trigger
  Function-Call Split/2 -> Function-Call Subsystem/Trigger
  Function-Call Split/1 -> Function-Call Subsystem1/Trigger
  DrvReportSetupData/1 -> Function-Call Subsystem1/1(In1)
  ISR100uProfiler/1 -> 100 usec Periodic profiler/Trigger
  Copy UART buffer/1(y) -> UartTxChar/1
  EnvGet/1 -> Function-Call Subsystem2/Trigger
  EnvSet/1 -> Function-Call Split/1
  UartGetChar/1 -> Copy UART buffer/Trigger
  DrvFeedback/1 -> Function-Call Subsystem/1(DrvFeedback1)
  ISR100uController/1 -> 100 usec Periodic controller/Trigger
  Function-Call Subsystem2/1(Out1) -> DrvCommand/1
  IdleLoopCAN/1 -> Idle process CAN interpreter/Trigger
  CanGetTxMsg/1 -> Get CAN Msg to transmit/Trigger
  Get CAN Msg to transmit/1(y) -> CanTxMsg/1
  SetupDrive/1 -> Drive configuration/Trigger
  RxMsg/1 -> CanSetRcvMsg/1(u)
  IdleLoopUART/1 -> Idle process UART interpreter/Trigger

== system HostOfSeal/Gft Servo Drive with SEAL/Drive sim/Speed estimator ==
  Encoder : Inport
  SpeedEstimae : Outport

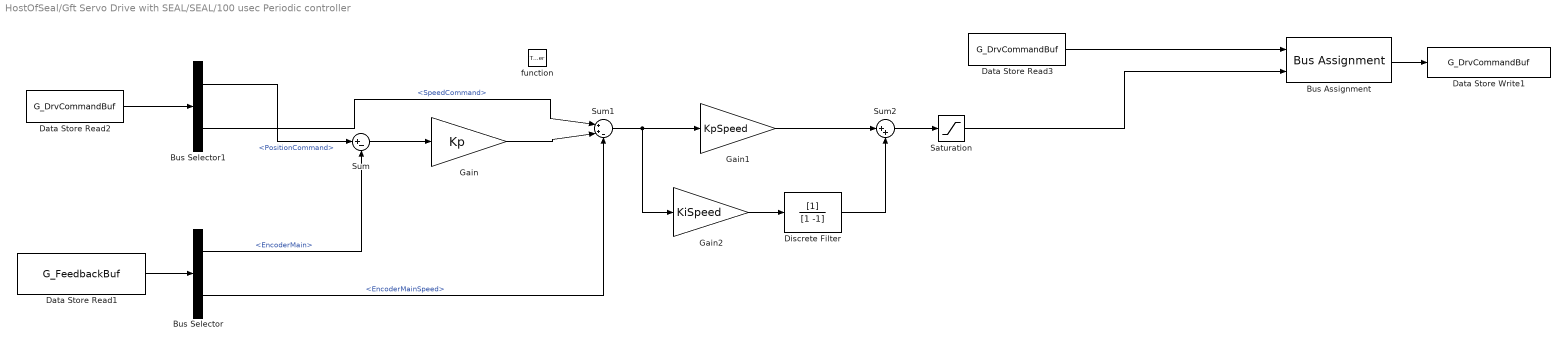
== system HostOfSeal/Gft Servo Drive with SEAL/SEAL/100 usec Periodic controller ==
  function : TriggerPort  TriggerType=function-call  VariantControl=(inherit)
  Bus Assignment : BusAssignment  AssignedSignals=CurrentCommand
  Bus Selector : BusSelector  OutputSignals=EncoderMain,EncoderMainSpeed
  Bus Selector1 : BusSelector  OutputSignals=PositionCommand,SpeedCommand
  Data Store Read1 : DataStoreRead  DataStoreName=G_FeedbackBuf  IndexOptions=Index vector (dialog)  Indices=1  OutputSizes=1
  Data Store Read2 : DataStoreRead  DataStoreName=G_DrvCommandBuf  IndexOptions=Index vector (dialog)  Indices=1  OutputSizes=1
  Data Store Read3 : DataStoreRead  DataStoreName=G_DrvCommandBuf  IndexOptions=Index vector (dialog)  Indices=1  OutputSizes=1
  Data Store Write1 : DataStoreWrite  DataStoreName=G_DrvCommandBuf  IndexOptions=Index vector (dialog)  Indices=1  OutputSizes=1
  Discrete Filter : DiscreteFilter  Denominator=[1 -1]
  Gain : Gain  Gain=Kp
  Gain1 : Gain  Gain=KpSpeed
  Gain2 : Gain  Gain=KiSpeed
  Saturation : Saturate
  Sum : Sum  Inputs=|+-
  Sum1 : Sum  Inputs=|++-
  Sum2 : Sum  Inputs=|++
  wires:
  Data Store Read3/1 -> Bus Assignment/1
  Bus Assignment/1 -> Data Store Write1/1
  Data Store Read1/1 -> Bus Selector/1
  Bus Selector/1 -> Sum/2  "<EncoderMain>"
  Data Store Read2/1 -> Bus Selector1/1
  Bus Selector1/1 -> Sum/1  "<PositionCommand>"
  Sum/1 -> Gain/1
  Gain/1 -> Sum1/2
  Bus Selector1/2 -> Sum1/1  "<SpeedCommand>"
  Bus Selector/2 -> Sum1/3  "<EncoderMainSpeed>"
  Sum1/1 -> Gain2/1, Gain1/1
  Gain2/1 -> Discrete Filter/1
  Gain1/1 -> Sum2/1
  Discrete Filter/1 -> Sum2/2
  Sum2/1 -> Saturation/1
  Saturation/1 -> Bus Assignment/2

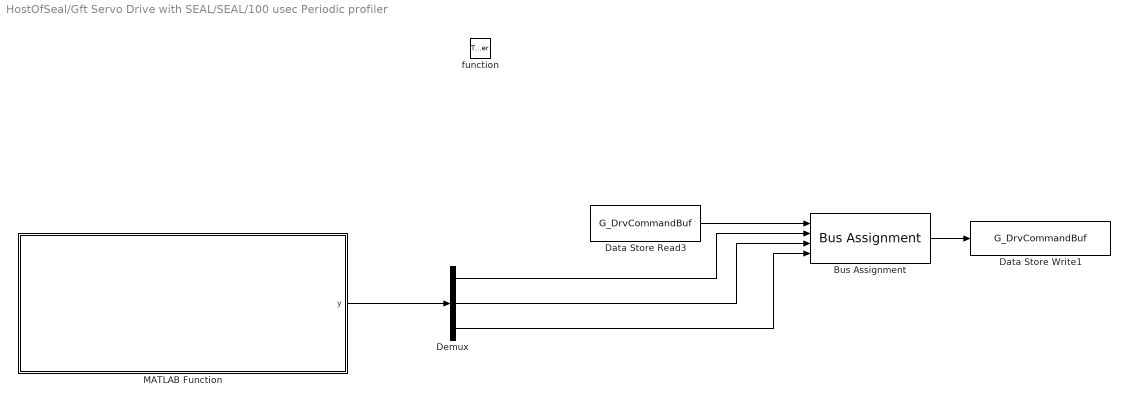
== system HostOfSeal/Gft Servo Drive with SEAL/SEAL/100 usec Periodic profiler ==
  function : TriggerPort  TriggerType=function-call  VariantControl=(inherit)
  Bus Assignment : BusAssignment  AssignedSignals=PositionCommand,SpeedCommand,CurrentCommand
  Data Store Read3 : DataStoreRead  DataStoreName=G_DrvCommandBuf  IndexOptions=Index vector (dialog)  Indices=1  OutputSizes=1
  Data Store Write1 : DataStoreWrite  DataStoreName=G_DrvCommandBuf  IndexOptions=Index vector (dialog)  Indices=1  OutputSizes=1
  Demux : Demux  Outputs=3
  MATLAB Function : MATLAB Function  TreatAsAtomicUnit=on
  wires:
  Data Store Read3/1 -> Bus Assignment/1
  MATLAB Function/1(y) -> Demux/1
  Demux/1 -> Bus Assignment/2
  Demux/2 -> Bus Assignment/3
  Demux/3 -> Bus Assignment/4
  Bus Assignment/1 -> Data Store Write1/1

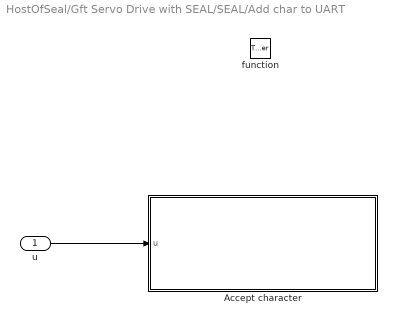
== system HostOfSeal/Gft Servo Drive with SEAL/SEAL/Add char to UART ==
  u : Inport  OutDataTypeStr=uint16  PortDimensions=1
  function : TriggerPort  TriggerType=function-call  VariantControl=(inherit)
  Accept character : MATLAB Function  TreatAsAtomicUnit=on
  wires:
  u/1 -> Accept character/1(u)

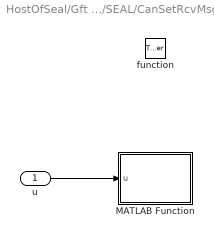
== system HostOfSeal/Gft Servo Drive with SEAL/SEAL/CanSetRcvMsg ==
  u : Inport  OutDataTypeStr=Bus: CANMessage_T
  function : TriggerPort  TriggerType=function-call  VariantControl=(inherit)
  MATLAB Function : MATLAB Function  TreatAsAtomicUnit=on
  wires:
  u/1 -> MATLAB Function/1(u)

== system HostOfSeal/Gft Servo Drive with SEAL/SEAL/Copy UART buffer ==
  function : TriggerPort  TriggerType=function-call  VariantControl=(inherit)
  Get From UART FIFO : MATLAB Function  TreatAsAtomicUnit=on
  y : Outport
  wires:
  Get From UART FIFO/1(y) -> y/1

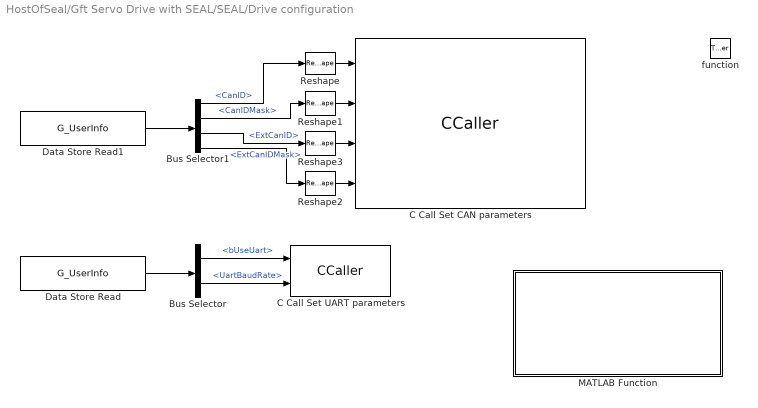
== system HostOfSeal/Gft Servo Drive with SEAL/SEAL/Drive configuration ==
  function : TriggerPort  TriggerType=function-call  VariantControl=(inherit)
  Bus Selector : BusSelector  OutputSignals=bUseUart,UartBaudRate
  Bus Selector1 : BusSelector  OutputSignals=CanID,CanIDMask,ExtCanID,ExtCanIDMask
  C Call Set CAN parameters : CCaller  FunctionName=SetCanParameters  PortSpecificationStruct="%)30     .    6 <   8    (     @         %    \"     0    !     0         %  0 \"0    $    _    07)G3F%M90  4&]R=$YA;64 4V-O<&4     26YD97@     5'EP90      4VEZ90      27-';&]B86P   X    X    !@    @    $          4    (     0    4    !         !     %    0V%N240    .    .     8    (    !          %    \"     $    %     0         0    !0   $-A;DE$    #@   #@    &    \"     0         !0    @    !   ...(+2149 chars)"
  C Call Set UART parameters : CCaller  FunctionName=SetUartParameters  PortSpecificationStruct="%)30     .    V ,   8    (     @         %    \"     (    !     0         %  0 \"0    $    _    07)G3F%M90  4&]R=$YA;64 4V-O<&4     26YD97@     5'EP90      4VEZ90      27-';&]B86P   X    X    !@    @    $          4    (     0    <    !         !     '    =7-E56%R=  .    .     8    (    !          %    \"     $    '     0         0    !P   '5S955A<G0 #@   #@    &    \"     0         !0    @    !    !0    $         $     4   !);G!U=     X    X    !@    @    &          4    (     0    $    !          D    (               .    .     8    (    !          %    \"     $    &     0         0    !@   '5I;G0Q-@  #@   #     &    \"     0         !0    @    !     0    $         $  ! #$    .    ,     8    (    \"0(        %    \"     $    !     0         \"  $       X    X    !@    @    $          4    (     0    @    !         !     (    8F%U9%)A=&4.    .     8    (    !          %    \"     $    (     0         0    \"    &)A=612871E#@   #@    &    \"     0         !0    @    !    !0    $         $     4   !);G!U=     X    X    !@    @    &          4    (     0    $    !          D    (            \\#\\.    .     8    (    !          %    \"     $    &     0         0    !@   '5I;G0S,@  #@   #     &    \"     0         !0    @    !     0    $         $  ! #$    .    ,     8    (    \"0(        %    \"     $    !     0         \"  $"
  Data Store Read : DataStoreRead  DataStoreName=G_UserInfo  IndexOptions=Index vector (dialog)  Indices=1  OutputSizes=1
  Data Store Read1 : DataStoreRead  DataStoreName=G_UserInfo  IndexOptions=Index vector (dialog)  Indices=1  OutputSizes=1
  MATLAB Function : MATLAB Function  TreatAsAtomicUnit=on
  Reshape{,1..3} (4 alike) : Reshape
  wires:
  Data Store Read/1 -> Bus Selector/1
  Bus Selector/1 -> C Call Set UART parameters/1  "<bUseUart>"
  Bus Selector/2 -> C Call Set UART parameters/2  "<UartBaudRate>"
  Data Store Read1/1 -> Bus Selector1/1
  Bus Selector1/1 -> Reshape/1  "<CanID>"
  Bus Selector1/2 -> Reshape1/1  "<CanIDMask>"
  Bus Selector1/4 -> Reshape2/1  "<ExtCanIDMask>"
  Reshape/1 -> C Call Set CAN parameters/1
  Reshape1/1 -> C Call Set CAN parameters/2
  Reshape2/1 -> C Call Set CAN parameters/4
  Bus Selector1/3 -> Reshape3/1  "<ExtCanID>"
  Reshape3/1 -> C Call Set CAN parameters/3

== system HostOfSeal/Gft Servo Drive with SEAL/SEAL/Function-Call Subsystem ==
  DrvFeedback1 : Inport
  function : TriggerPort  TriggerType=function-call  VariantControl=(inherit)
  Driver feedback interface : DataStoreWrite  DataStoreName=G_FeedbackBuf  IndexOptions=Index vector (dialog)  Indices=1  OutputSizes=1
  wires:
  DrvFeedback1/1 -> Driver feedback interface/1

== system HostOfSeal/Gft Servo Drive with SEAL/SEAL/Function-Call Subsystem1 ==
  In1 : Inport
  function : TriggerPort  TriggerType=function-call  VariantControl=(inherit)
  Data Store Write : DataStoreWrite  DataStoreName=G_SetupReportBuf  IndexOptions=Index vector (dialog)  Indices=1  OutputSizes=1
  wires:
  In1/1 -> Data Store Write/1

== system HostOfSeal/Gft Servo Drive with SEAL/SEAL/Function-Call Subsystem2 ==
  function : TriggerPort  TriggerType=function-call  VariantControl=(inherit)
  Driver command interface : DataStoreRead  DataStoreName=G_DrvCommandBuf  IndexOptions=Index vector (dialog)  Indices=1  OutputSizes=1
  Out1 : Outport
  wires:
  Driver command interface/1 -> Out1/1

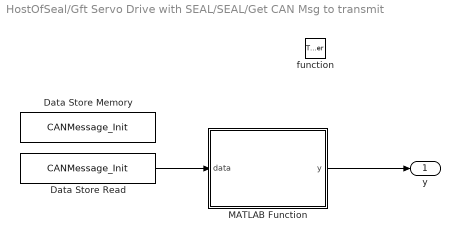
== system HostOfSeal/Gft Servo Drive with SEAL/SEAL/Get CAN Msg to transmit ==
  function : TriggerPort  TriggerType=function-call  VariantControl=(inherit)
  Data Store Memory : DataStoreMemory  DataStoreName=CANMessage_Init  WriteAfterWriteMsg=warning  ShowAdditionalParam=off  OutDataTypeStr=Bus: CANMessage_T
  Data Store Read : DataStoreRead  DataStoreName=CANMessage_Init  IndexOptions=Index vector (dialog)  Indices=1  OutputSizes=1
  MATLAB Function : MATLAB Function  TreatAsAtomicUnit=on
  y : Outport
  wires:
  MATLAB Function/1(y) -> y/1
  Data Store Read/1 -> MATLAB Function/1(data)

== system HostOfSeal/Gft Servo Drive with SEAL/SEAL/Idle process CAN interpreter ==
  function : TriggerPort  TriggerType=function-call  VariantControl=(inherit)
  CAN message response : MATLAB Function  TreatAsAtomicUnit=on

== system HostOfSeal/Gft Servo Drive with SEAL/SEAL/Idle process UART interpreter ==
  function : TriggerPort  TriggerType=function-call  VariantControl=(inherit)
  G_MicroInterp : DataStoreMemory  DataStoreName=G_MicroInterp  WriteAfterWriteMsg=warning  ShowAdditionalParam=off  OutDataTypeStr=Bus: MicroInterp_T  StateMustResolveToSignalObject=on
      settings: LockScale=on
  UART message response : MATLAB Function  TreatAsAtomicUnit=on

== matlab function HostOfSeal/Gft Servo Drive with SEAL/SEAL/Idle process CAN interpreter/CAN message response ==
  data: G_pCANCyclicBuf_in data_store_memory; G_pCANCyclicBuf_out data_store_memory
function OutBuf



global G_pCANCyclicBuf_in  
global G_pCANCyclicBuf_out  

if (G_pCANCyclicBuf_in.PutCounter == G_pCANCyclicBuf_in.FetchCounter ) 
    return ; 
end

for cnt = 1:3 
% The CAN queues count like C (zero based), yet the code here is matlab (1
% based) so we have to increment the counters to be valid Matlab indices
    nfetch  = bitand( G_pCANCyclicBuf_in.FetchCounter ,63 ) + 1; 
    nput    = bitand( G_pCANCyclicBuf_out.PutCounter  , 63) + 1 ; 
    nextput = bitand( nput + 1 , 63)  ;  
    if ( nextput == G_pCANCyclicBuf_out.FetchCounter) 
        break ; % Output queue is full 
    end 

    nmsgGet     = nfetch * 2 - 1 ; 
    nmsgPut     = nput  * 2 -  1 ; 
    nextmsg     = G_pCANCyclicBuf_in.CANQueue([nmsgGet,nmsgGet+1]) ;

    nextid      = G_pCANCyclicBuf_in.CANID(nfetch) ; 
    nextattrib  = G_pCANCyclicBuf_in.DLenAndAttrib(nfetch) ; 

    % Idiotic interpreter - just return what it got 
    G_pCANCyclicBuf_out.CANQueue([nmsgPut,nmsgPut+1]) = nextmsg; 
    G_pCANCyclicBuf_out.CANID(nput) = nextid ; 
    G_pCANCyclicBuf_out.DLenAndAttrib(nput) = nextattrib ;

    % Update TX and RX counters
    G_pCANCyclicBuf_out.PutCounter  = nextput ;
    G_pCANCyclicBuf_in.FetchCounter = bitand( nfetch + 1  , 63) ; 

    if (G_pCANCyclicBuf_in.PutCounter == G_pCANCyclicBuf_in.FetchCounter ) 
        break ; 
    end
end


end
% celems(1) = SetBusElement('PutCounter','uint16',"The place in the CANQueue where the next message is to be put" ) ; 
% celems(2) = SetBusElement('FetchCounter','uint16',"The location in the CANQueue of the next message to read" ) ; 
% celems(3) = SetBusElement('CANError','uint16',"CAN error" ) ; 
% celems(4) = SetBusElement('CANQueue','uint32',"Software Queue for incoming UART characters" ,[64,2]) ; 
% celems(5) = SetBusElement('TxFetchCounter','uint16',"The location in the CANQueue of the next message to transmit" ) ; 
% celems(6) = SetBusElement('CANID','uint32',"Can ID, 11 or 29bit" ,[64,1]) ; 
% celems(7) = SetBusElement('DLenAndAttrib','uint16',"Data length and attributes" ,[64,1]) ;
